simulink model "magnet_force"  (R2018a)
settings: Solver=VariableStepAuto  StartTime=0.0  StopTime=10.0  RelTol=1e-3
settings Model: Creator=saad  LastModifiedBy=saad

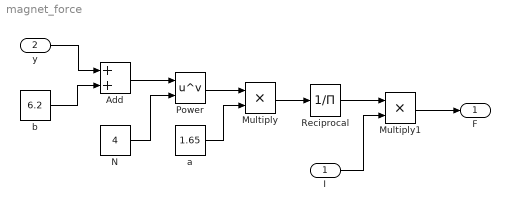
== system magnet_force ==
  I : Inport
  y : Inport  Port=2
  Add : Sum
  Multiply : Product
  Multiply1 : Product
  N : Constant  Value=4
  Power : Math  Operator=pow  SaturateOnIntegerOverflow=on
  Reciprocal : Product  Inputs=/
  a : Constant  Value=1.65
  b : Constant  Value=6.2
  F : Outport
  wires:
  y/1 -> Add/1
  I/1 -> Multiply1/2
  b/1 -> Add/2
  Power/1 -> Multiply/1
  Add/1 -> Power/1
  Reciprocal/1 -> Multiply1/1
  a/1 -> Multiply/2
  Multiply/1 -> Reciprocal/1
  N/1 -> Power/2
  Multiply1/1 -> F/1
